simulink library "cct"  (Simulink 8.1)
settings: Solver=ode1  StartTime=0.0  StopTime=Inf  FixedStep=0.001  RelTol=1e-3
PostLoadFcn:
  | , if any(exist('dsrtsu_mdlpostloadfcn', 'file') == [2, 3, 6]), try dsrtsu_mdlpostloadfcn('Execute', bdroot); catch fprintf('Error in PostLoadFcn (dsrtsu_mdlpostloadfcn) for model "%s":\n %s\n', bdroot, lasterr); end, end,
libraries: cctc x1, cctd x1
settings Model: DSRTSU_INTERNAL_RTI_VER=450  DSRTSU_INTERNAL_RTI_TYPE=rti1401  RTICANMMDATA=struct('GeneralSetupData',struct('modelroot','D:\ELN150201_TAIWAN\trunk\AdasDragon\software\sw_development\arch\app\jud','generalsettings',struct('filesettings',struct('destfolder',struct('Name','RTICANMM_FILES','Check',1),'buildfolder',struct('Name','.','Check',1),'AbsDestfolder',struct('Name','D:\ELN150201_TAIWAN\trunk\AdasDragon\software\sw_development\arch\app\jud\RTICANMM_FILES'),'AbsBuildfolder',struct('Name','D:\ELN150201_TAIWAN\trunk\AdasDragon\software\sw_development\arch\app\jud'))),'options',struct('addpaths',1,'rmpaths',1,'addtrcexclusion',logical(1),'cannavigator',struct('checkmonitoring',0),'show_usrtrc',0,'use_usrtrc',0),'advanced',struct('options',[1 1 1 1 1 1 1 1 1 1 1 1 1 1 1 1 1 1 1 1 1 1 1 1 1 1 1 1 1 1 1 1 1 1 1 1 1 1 1 1 1 1 1 1 1 1 1 1 1 1 1 1 1 1 1 1 1 1 1 1 1 1 1 1 1 1 1 1 1 1 1 1 1 1 1 1 1 1 1 1 1 1 1 1 1 1 1 1 1 1 1 1 1 1 1 1 1 1 1 1]),'MPSetup',{{}},'modelname','cct','block','cct'))  DSRTSU_INTERNAL_RTIFPGA=40  Creator=AT015411  LastModifiedBy=AT015555

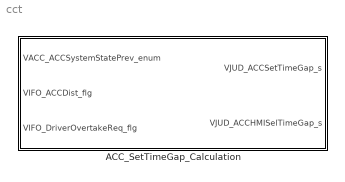
== system cct ==
  ACC_SetTimeGap_Calculation : Subsystem

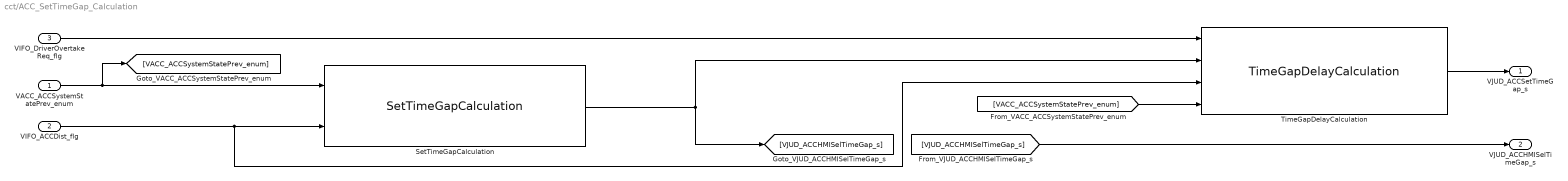
== system cct/ACC_SetTimeGap_Calculation ==
  VACC_ACCSystemStatePrev_enum : Inport
  VIFO_ACCDist_flg : Inport  Port=2
  VIFO_DriverOvertakeReq_flg : Inport  Port=3
  SetTimeGapCalculation : cctc/SetTimeGapCalculation
  TimeGapDelayCalculation : cctd/TimeGapDelayCalculation
  VJUD_ACCSetTimeGap_s : Outport
  VJUD_ACCHMISelTimeGap_s : Outport  Port=2
  wires:
  VIFO_DriverOvertakeReq_flg/1 -> TimeGapDelayCalculation/1
  VACC_ACCSystemStatePrev_enum/1 -> SetTimeGapCalculation/1, [VACC_ACCSystemStatePrev_enum]
  VIFO_ACCDist_flg/1 -> TimeGapDelayCalculation/3, SetTimeGapCalculation/2
  SetTimeGapCalculation/1 -> TimeGapDelayCalculation/2, [VJUD_ACCHMISelTimeGap_s]
  TimeGapDelayCalculation/1 -> VJUD_ACCSetTimeGap_s/1
  [VACC_ACCSystemStatePrev_enum] -> TimeGapDelayCalculation/4
  [VJUD_ACCHMISelTimeGap_s] -> VJUD_ACCHMISelTimeGap_s/1
